simulink model "case1_mdl"  (Simulink 5.0)
settings: Solver=ode45  StartTime=0.0  StopTime=3999  RelTol=1e-3
undefined symbols (not defined in the file or in its folder): Ts
settings Model: Creator=kannan  LastModifiedBy=kannan  ExtModeAutoUpdateStatusClock=off

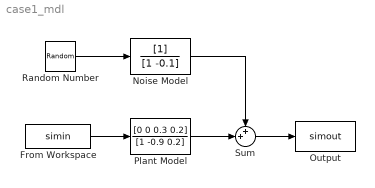
== system case1_mdl ==
  From Workspace : FromWorkspace  VariableName=simin  SampleTime=Ts
  Noise Model : DiscreteFilter  Denominator=[1 -0.1]  SampleTime=Ts
  Output : ToWorkspace  VariableName=simout  SampleTime=Ts  SaveFormat=Array
  Plant Model : DiscreteFilter  Numerator=[0 0 0.3 0.2]  Denominator=[1 -0.9 0.2]  SampleTime=Ts
  Random Number : RandomNumber  Variance=0.2  SampleTime=Ts
  Sum : Sum  Inputs=++|  SaturateOnIntegerOverflow=on
  wires:
  Random Number/1 -> Noise Model/1
  From Workspace/1 -> Plant Model/1
  Noise Model/1 -> Sum/1
  Plant Model/1 -> Sum/2
  Sum/1 -> Output/1
